simulink model "BPM_Sfun_Open_Loop"  (R2022b)
settings: configuration reference "ModelConfig_var" (kept outside this file)
undefined symbols (not defined in the file or in its folder): TimeSteps
settings Model: Creator=BEDNASA  LastModifiedBy=BEDNASA
settings ConfigSetRef: SourceName=ModelConfig_var  SourceLocation=Base Workspace

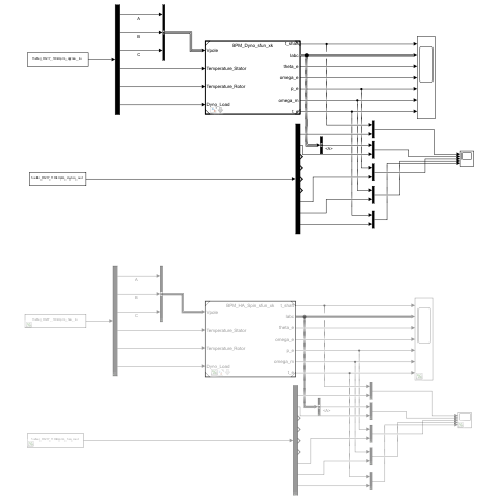
[thumbnail: Simulink's stored preview of the top-level diagram]
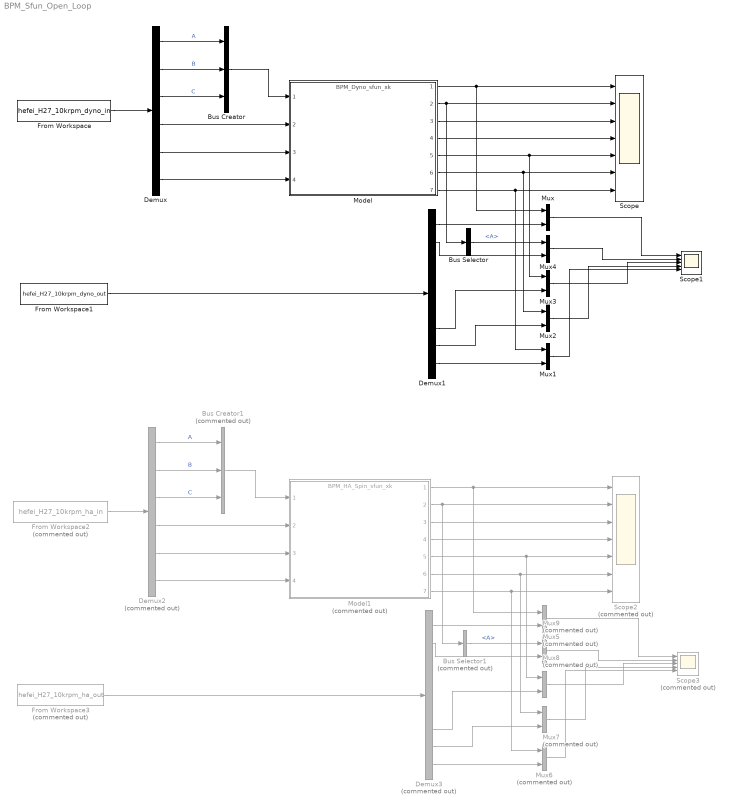
== system BPM_Sfun_Open_Loop ==
  Bus Creator : BusCreator  Inputs=3  OutDataTypeStr=Bus: XabcBus
  Bus Creator1 : BusCreator  Commented=on  Inputs=3  OutDataTypeStr=Bus: XabcBus
  Bus Selector : BusSelector  OutputSignals=A
  Bus Selector1 : BusSelector  Commented=on  OutputSignals=A
  Demux : Demux  Outputs=6
  Demux1 : Demux  Outputs=9
  Demux2 : Demux  Commented=on  Outputs=6
  Demux3 : Demux  Commented=on  Outputs=9
  From Workspace : FromWorkspace  VariableName=hefei_H27_10krpm_dyno_in
  From Workspace1 : FromWorkspace  VariableName=hefei_H27_10krpm_dyno_out  SampleTime=TimeSteps.ModelStep
  From Workspace2 : FromWorkspace  Commented=on  VariableName=hefei_H27_10krpm_ha_in
  From Workspace3 : FromWorkspace  Commented=on  VariableName=hefei_H27_10krpm_ha_out  SampleTime=TimeSteps.ModelStep
  Model : ModelReference  ModelNameDialog=BPM_Dyno_sfun_xk  UsingDefaultArgumentValue=0,0,0,0,0,0,0,0,0,0,0,0,0,0,0,0,0,0,0,0,0,0,0,0,0,0,0,0,0,0,0,0,0,0,0,0,0,0,0,0,0,0,0,0,0,0,0,0,0,0,0  SimulationMode=Normal  ModelReferenceVersion=10.3  bpm_Rs_0=Motor_prm.Electrical.Rs_0  bpm_Ld_0=Motor_prm.Electrical.Ld_0  bpm_Lq_0=Motor_prm.Electrical.Lq_0  bpm_PM_flux_h1_0=Motor_prm.Electrical.PM_flux_h1_0  bpm_NPP=Motor_prm.Electrical.NPP  bpm_Jrotor=Motor_prm.Mechanical.Jrotor  bpm_B=Motor_prm.Mechanical.B  bpm_TR=Motor_prm.Mechanical.TR  bpm_Temp_stator_0=Motor_prm.Thermal.Temp_stator_0  bpm_Temp_rotor_0=Motor_prm.Thermal.Temp_rotor_0  bpm_Rs_stator_alpha=Motor_prm.Thermal.Rs_alpha  bpm_PM_rotor_alpha=Motor_prm.Thermal.PM_alpha  bpm_Ls_sat_flag=1  bpm_Loss_flag=1  bpm_Loss_th=10  bpm_Rsa_aux=0  bpm_Rsb_aux=0  bpm_Rsc_aux=0  Mech_HAs_J_drum=0  Mech_HAs_damp=0  Mech_HAs_m_unb=0  Mech_HAs_r_unb=0  Mech_HAs_TR=0  Mech_HAs_CF=0  Mech_VAa_water_vol=0  Mech_VAa_imp_dens=0  Mech_VAa_gear_ratio=0  Mech_VAa_clothes_mass=0  Mech_VAa_belt_ratio=0  Mech_VAa_basket_dia=0  Mech_VAa_basket_dens=0  Mech_VAa_J_basket=0  Mech_VAa_J_impeller=0  Mech_VAs_m_u=0  Mech_VAs_m_t=0  Mech_VAs_m_d=0  Mech_VAs_m_b1=0  Mech_VAs_m_b2=0  Mech_VAs_e=0  Mech_VAs_d=0  Mech_VAs_belt_rat=0  Mech_VAs_T_f=0  Mech_VAs_K=0  Mech_VAs_I_zt=0  Mech_VAs_D_r=0  SimulationMode=Normal
  Model1 : ModelReference  Commented=on  ModelNameDialog=BPM_HA_Spin_sfun_xk  UsingDefaultArgumentValue=0,0,0,0,0,0,0,0,0,0,0,0,0,0,0,0,0,0,0,0,0,0,0,0,0,0,0,0,0,0,0,0,0,0,0,0,0,0,0,0,0,0,0,0,0,0,0,0,0,0,0  SimulationMode=Normal  ModelReferenceVersion=10.11  bpm_Rs_0=Motor_prm.Electrical.Rs_0  bpm_Ld_0=Motor_prm.Electrical.Ld_0  bpm_Lq_0=Motor_prm.Electrical.Lq_0  bpm_PM_flux_h1_0=Motor_prm.Electrical.PM_flux_h1_0  bpm_NPP=Motor_prm.Electrical.NPP  bpm_Jrotor=Motor_prm.Mechanical.Jrotor  bpm_B=Motor_prm.Mechanical.B  bpm_TR=Motor_prm.Mechanical.TR  bpm_Temp_stator_0=Motor_prm.Thermal.Temp_stator_0  bpm_Temp_rotor_0=Motor_prm.Thermal.Temp_rotor_0  bpm_Rs_stator_alpha=Motor_prm.Thermal.Rs_alpha  bpm_PM_rotor_alpha=Motor_prm.Thermal.PM_alpha  bpm_Ls_sat_flag=1  bpm_Loss_flag=1  bpm_Loss_th=10  bpm_Rsa_aux=0  bpm_Rsb_aux=0  bpm_Rsc_aux=0  Mech_HAs_J_drum=Mechanical.JDrum  Mech_HAs_damp=Mechanical.damp  Mech_HAs_m_unb=Mechanical.m_unb  Mech_HAs_r_unb=Mechanical.r_unb  Mech_HAs_TR=Motor_prm.Mechanical.TR  Mech_HAs_CF=0  Mech_VAa_water_vol=0  Mech_VAa_imp_dens=0  Mech_VAa_gear_ratio=0  Mech_VAa_clothes_mass=0  Mech_VAa_belt_ratio=0  Mech_VAa_basket_dia=0  Mech_VAa_basket_dens=0  Mech_VAa_J_basket=0  Mech_VAa_J_impeller=0  Mech_VAs_m_u=0  Mech_VAs_m_t=0  Mech_VAs_m_d=0  Mech_VAs_m_b1=0  Mech_VAs_m_b2=0  Mech_VAs_e=0  Mech_VAs_d=0  Mech_VAs_belt_rat=0  Mech_VAs_T_f=0  Mech_VAs_K=0  Mech_VAs_I_zt=0  Mech_VAs_D_r=0  SimulationMode=Normal
  Mux{,1..4} (5 alike) : Mux  Inputs=2
  Mux{5..9} (5 alike) : Mux  Commented=on  Inputs=2
  Scope : Scope  NumInputPorts=7
  Scope1 : Scope  NumInputPorts=5
  Scope2 : Scope  Commented=on  NumInputPorts=7
  Scope3 : Scope  Commented=on  NumInputPorts=5
  wires:
  From Workspace/1 -> Demux/1
  Demux/6 -> Model/4
  Demux/5 -> Model/3
  Demux/4 -> Model/2
  Bus Creator/1 -> Model/1
  Demux/1 -> Bus Creator/1  "A"
  Demux/2 -> Bus Creator/2  "B"
  Demux/3 -> Bus Creator/3  "C"
  Model/1 -> Mux/1, Scope/1
  Model/2 -> Bus Selector/1, Scope/2
  Model/3 -> Scope/3
  Model/4 -> Scope/4
  Model/5 -> Scope/5, Mux3/1
  Model/6 -> Mux2/1, Scope/6
  Model/7 -> Mux1/1, Scope/7
  From Workspace1/1 -> Demux1/1
  Demux1/1 -> Mux/2
  Demux1/9 -> Mux1/2
  Demux1/8 -> Mux2/2
  Demux1/7 -> Mux3/2
  Demux1/2 -> Mux4/2
  Mux/1 -> Scope1/1
  Mux4/1 -> Scope1/2
  Mux3/1 -> Scope1/3
  Mux2/1 -> Scope1/4
  Mux1/1 -> Scope1/5
  Bus Selector/1 -> Mux4/1  "<A>"
  Demux3/7 -> Mux8/2
  Mux9/1 -> Scope3/2
  Demux3/9 -> Mux6/2
  Demux3/8 -> Mux7/2
  Demux3/2 -> Mux9/2
  Mux5/1 -> Scope3/1
  Mux8/1 -> Scope3/3
  Model1/2 -> Bus Selector1/1, Scope2/2
  Model1/7 -> Mux6/1, Scope2/7
  Model1/4 -> Scope2/4
  Model1/6 -> Mux7/1, Scope2/6
  From Workspace3/1 -> Demux3/1
  Bus Selector1/1 -> Mux9/1  "<A>"
  Mux7/1 -> Scope3/4
  Mux6/1 -> Scope3/5
  From Workspace2/1 -> Demux2/1
  Demux2/1 -> Bus Creator1/1  "A"
  Model1/3 -> Scope2/3
  Demux2/6 -> Model1/4
  Bus Creator1/1 -> Model1/1
  Model1/1 -> Mux5/1, Scope2/1
  Model1/5 -> Scope2/5, Mux8/1
  Demux2/2 -> Bus Creator1/2  "B"
  Demux2/5 -> Model1/3
  Demux2/4 -> Model1/2
  Demux3/1 -> Mux5/2
  Demux2/3 -> Bus Creator1/3  "C"
